simulink model "MDCC_DeadComp"  (R2023a)
settings: Solver=FixedStepDiscrete  StartTime=0.0  StopTime=10.0  FixedStep=0.0001  RelTol=1e-3
model workspace (MATLAB code in the model file):
  | cmdLim = Simulink.Parameter;
  | cmdLim.Value = 15;
  | cmdLim.Description = 'Limit for controlling the maximum surface command angle.';
  | cmdLim.Min = 0;
  | cmdLim.Max = 90;
  | cmdLim.DocUnits = 'deg';
  | 
  | dispGain = Simulink.Parameter;
  | dispGain.Value = 0.75;
  | dispGain.Description = 'Gain applied to the displacement error.';
  | dispGain.Min = 0;
  | dispGain.Max = [];
  | dispGain.DocUnits = 'deg/sec/deg';
  | 
  | dispLim = Simulink.Parameter;
  | dispLim.Value = 30;
  | dispLim.Description = 'Limit for controlling the maximum commanded angle.';
  | dispLim.Min = 0;
  | dispLim.Max = 180;
  | dispLim.DocUnits = 'deg';
  | 
  | intGain = Simulink.Parameter;
  | intGain.Value = 0.5;
  | intGain.Description = 'Gain applied to the integral error.';
  | intGain.Min = 0;
  | intGain.Max = [];
  | intGain.DocUnits = 'deg/sec/deg/sec';
  | 
  | intLim = Simulink.Parameter;
  | intLim.Value = 5;
  | intLim.Description = 'Limit for controlling the maximum commanded angle.';
  | intLim.Min = 0;
  | intLim.Max = 90;
  | intLim.DocUnits = 'deg';
  | 
  | rateGain = Simulink.Parameter;
  | rateGain.Value = 2;
  | rateGain.Description = 'Gain applied to the rate error.';
  | rateGain.Min = 0;
  | rateGain.Max = [];
  | rateGain.DocUnits = 'deg/deg/sec';
  | 
  | rateLim = Simulink.Parameter;
  | rateLim.Value = 6;
  | rateLim.Description = 'Limit for controlling the maximum commanded angle.';
  | rateLim.Min = 0;
  | rateLim.Max = 180;
  | rateLim.DocUnits = 'deg/sec';
  | 
  | hdgGain = Simulink.Parameter;
  | hdgGain.Value = 0.015;
values from neighbouring files (symbols this model uses):
  Ts = 5E-6    (= 5e-06)    [iPMSM_data.m]
undefined symbols (not defined in the file or in its folder): CosTable12bit_Y, GLBCal_GLBCal_Kf_DCLinkOverVolErrThd_V, GLBCal_GLBCal_Kf_DCLinkUnderVolErrThd_V, GLBCal_GLBCal_Kf_EquiLd_NULL, GLBCal_GLBCal_Kf_EquiLq_NULL, GLBCal_GLBCal_Kf_MotorRatedSpeed_rpm, GLBCal_GLBCal_Kf_MotorSpeedHysteresis_Coef, GLBCal_Ke_MotorPolePairsNum_NULL, IoHwAbOpArg_PwmDutyCyclePhU_NULL, IoHwAbOpArg_PwmDutyCyclePhV_NULL, IoHwAbOpArg_PwmDutyCyclePhW_NULL, IoHwAbOpArg_PwmOutputEn, KbMDCC_DeadTimeCompEn_flg, KbMDCC_MCF_flgHarmInject_flg, KbMDCC_SetEAngleEn_flg, KbMDCC_UdUqFwOmit_flg, KfMDCC_AbsIs_A, KfMDCC_ActiveDischargeIdCurVal_A, KfMDCC_ActiveDischargeIqCurVal_A, KfMDCC_DCLinkVolRate_coef, KfMDCC_DeadRate_NULL, KfMDCC_DebugEAngleInit_rad, KfMDCC_DebugUalphaVolCmd_V, KfMDCC_DebugUbetaVolCmd_V, KfMDCC_DebugUdCmd_V, KfMDCC_DebugUqCmd_V, KfMDCC_DebugUsCmd_V, KfMDCC_DebugUsRate_V, KfMDCC_Duty_Coef, KfMDCC_IMCResp_NULL, KfMDCC_IMCStab_NULL, KfMDCC_InvParkCpPeriodTimesT_NULL, KfMDCC_MCF_Harm1113FLParamSpeedThrd_rads, KfMDCC_MCF_Harm57FLParamSpeedThrd_rads, KfMDCC_MCF_HarmCpnAg_NULL, KfMDCC_MCF_HarmfLParaHigh_coef, KfMDCC_MCF_HarmfLParaLow_coef, KfMDCC_MCF_HarmInSpdLimt_rpm, KfMDCC_MCF_HarmInUAlphaMax_V, KfMDCC_MCF_HarmInUbetaMax_V, KfMDCC_MotorSpeedRadsDAQFactor_NULL, KfMDCC_ResScal_Coef, KfMDCC_SelfHeatingUdVal_V, KfMDCC_SelfHeatingUdValRate_V, KfMDCC_SpdIMCResp_rpm, KfMDCC_SpdIMCStab_rpm, KfMDCC_VfMDCC_DCLinkCurValFactor_NULL, KfMDCM_DCLinkCoef, KfMDCM_DCLinkRatedVoltage_V, KfMDCM_FluxWeakningVolFWOffset_V, KuMDCC_PositionResolution_NULL, KuMDCC_SetEAngle_Null, MDSM_MCUStatus, PiIoHwSetInvState_C_Sws_UVW_PwmEnOutput, PiIoHwSetInvState_C_SwsSet_DPO_UVW_Asc, PiIoHwSetInvState_C_SwsSet_DPO_UVW_FW, PiIoHwSetPwmDuty_C_SwsSet_DPO_UVW_Duty, SinTable12bit_Y, SVPWM, VfMDCC_DeadComSpeedHigh_Rpm ... (+5)
libraries: simulink x14, PMSM_Library x4
(part 4 of 6)

== system MDCC_DeadComp/DoCurCtr_sys/MDCC/SVM_Calc/MDSA/SVPWM1/vIntp_PWMFOC_CalSec/CalVaVbVc ==
  Bus_UalphaUbeta : Inport
  Bus Creator : BusCreator  Inputs=3
  CalVa : Subsystem
  CalVb : Subsystem
  CalVc : Subsystem
  Bus_Vabc : Outport
  wires:
  Bus_UalphaUbeta/1 -> CalVc/1(In1), CalVb/1(In1), CalVa/1(In1)
  CalVb/1(Vb) -> Bus Creator/2  "Vb"
  CalVc/1(Vc) -> Bus Creator/3  "Vc"
  CalVa/1(Va) -> Bus Creator/1  "Va"
  Bus Creator/1 -> Bus_Vabc/1

== system MDCC_DeadComp/DoCurCtr_sys/MDCC/SVM_Calc/MDSA/SVPWM1/vIntp_PWMFOC_CalTriCompValue/CalCMPValue ==
  Bus_Tabc_IN : Inport
  N_VALUE_IN : Inport  Port=2
  Merge : Merge  Inputs=6
  Sec1 : Subsystem
  Sec2 : Subsystem
  Sec3 : Subsystem
  Sec4 : Subsystem
  Sec5 : Subsystem
  Sec6 : Subsystem
  Switch Case : SwitchCase  CaseConditions={1,2,3,4,5,6}  ShowDefaultCase=off
  Bus_CMP : Outport
  wires:
  N_VALUE_IN/1 -> Switch Case/1
  Bus_Tabc_IN/1 -> Sec2/1(Bus_Tabc_IN), Sec4/1(Bus_Tabc_IN), Sec6/1(Bus_Tabc_IN), Sec5/1(Bus_Tabc_IN), Sec3/1(Bus_Tabc_IN), Sec1/1(Bus_Tabc_IN)
  Merge/1 -> Bus_CMP/1
  Switch Case/1 -> [sec1]
  Switch Case/2 -> [sec2]
  Switch Case/3 -> [sec3]
  Switch Case/4 -> [sec4]
  Switch Case/5 -> [sec5]
  Switch Case/6 -> [sec6]
  [sec1] -> Sec1/Action
  [sec2] -> Sec2/Action
  [sec3] -> Sec3/Action
  [sec4] -> Sec4/Action
  [sec5] -> Sec5/Action
  [sec6] -> Sec6/Action
  Sec4/1(Bus_CMP) -> Merge/4
  Sec3/1(Bus_CMP) -> Merge/3
  Sec5/1(Bus_CMP) -> Merge/5
  Sec2/1(Bus_CMP) -> Merge/2
  Sec6/1(Bus_CMP) -> Merge/6
  Sec1/1(Bus_CMP) -> Merge/1

== system MDCC_DeadComp/DoCurCtr_sys/MDCC/SVM_Calc/MDSA/SVPWM1/vIntp_PWMFOC_CalTriCompValue/CalTabc ==
  Bus_XYZ_IN : Inport
  Bus_Ts_Vdc : Inport  Port=2
  N_VALUE_IN : Inport  Port=3
  Cal_T1T2 : Subsystem
  Cal_TabcValue : Subsystem
  Bus_Tabc : Outport
  wires:
  Bus_Ts_Vdc/1 -> Cal_TabcValue/2(Bus_Ts_Vdc)
  Bus_XYZ_IN/1 -> Cal_T1T2/1(Bus_XYZ_IN)
  N_VALUE_IN/1 -> Cal_T1T2/2(N_VALUE_IN)
  Cal_T1T2/1(Bus_T1T2_OUT) -> Cal_TabcValue/1(Bus_T1T2_IN)
  Cal_TabcValue/1(Bus_Tabc) -> Bus_Tabc/1

== system MDCC_DeadComp/DoCurCtr_sys/MDCC/SVM_Calc/MDSA/SVPWM1/vIntp_PWMFOC_CalTriCompValue/CalXYZ ==
  Bus_UalphaUbeta : Inport
  Bus_Ts_Vdc : Inport  Port=2
  Bus Creator : BusCreator  Inputs=3
  Cal_X : Subsystem
  Cal_Y : Subsystem
  Cal_Z : Subsystem
  BUS_XYZ : Outport
  wires:
  Bus_UalphaUbeta/1 -> Cal_Z/1(Bus_UalphaUbeta), Cal_Y/1(Bus_UalphaUbeta), Cal_X/1(Bus_UalphaUbeta)
  Cal_Y/1(Y_Value) -> Bus Creator/2  "Y"
  Cal_X/1(X_Value) -> Bus Creator/1  "X"
  Cal_Z/1(Z_Value) -> Bus Creator/3  "Z"
  Bus Creator/1 -> BUS_XYZ/1
  Bus_Ts_Vdc/1 -> Cal_Z/2(Bus_Ts_Vdc), Cal_X/2(Bus_Ts_Vdc), Cal_Y/2(Bus_Ts_Vdc)

== system MDCC_DeadComp/DoCurCtr_sys/MDCC/UdUqCalc_Sys/MDCC_MCF_Sys1/Enabled Subsystem/Harmonic_Injection_11/Subsystem ==
  MCF_Harm_isdDes11 : Inport
  MCF_Harm_isqDes11 : Inport  Port=2
  MCF_Harm_isdAct11 : Inport  Port=3
  MCF_Harm_isqAct11 : Inport  Port=4
  MCF_Sin11Ag : Inport  Port=5
  MCF_Cos11Ag : Inport  Port=6
  MCF_flgHarm11PIRest : Inport  Port=7
  MCF_Harm11_Kp : Inport  Port=8
  MCF_Harm11_Ki : Inport  Port=9
  ZeroEnable : EnablePort  StatesWhenEnabling=reset
  Harm_11Step_KpKi : Subsystem
  RevPark : Subsystem
  MCF_uAlpha_Harm11 : Outport  VectorParamsAs1DForOutWhenUnconnected=off
  MCF_uBeta_Harm11 : Outport  Port=2  VectorParamsAs1DForOutWhenUnconnected=off
  wires:
  MCF_Harm_isqDes11/1 -> Harm_11Step_KpKi/2(MCF_Harm_isqDes11)  "MCF_Harm_isqDes11"
  MCF_Harm_isqAct11/1 -> Harm_11Step_KpKi/4(MCF_Harm_isqAct11)
  RevPark/2(MCF_uBeta_Harm11) -> MCF_uBeta_Harm11/1
  MCF_Harm_isdAct11/1 -> Harm_11Step_KpKi/3(MCF_Harm_isdAct11)
  RevPark/1(MCF_uAlpha_Harm11) -> MCF_uAlpha_Harm11/1
  MCF_Harm_isdDes11/1 -> Harm_11Step_KpKi/1(MCF_Harm_isdDes11)  "MCF_Harm_isdDes11"
  MCF_flgHarm11PIRest/1 -> Harm_11Step_KpKi/5(MCF_flgHarm11PIRest)
  Harm_11Step_KpKi/1(MCF_Harm_ud11PI) -> RevPark/1(MCF_Harm_ud11PI)
  Harm_11Step_KpKi/2(MCF_Harm_uq11PI) -> RevPark/2(MCF_Harm_uq11PI)
  MCF_Sin11Ag/1 -> RevPark/3(MCF_Sin11Ag)
  MCF_Cos11Ag/1 -> RevPark/4(MCF_Cos11Ag)
  MCF_Harm11_Kp/1 -> Harm_11Step_KpKi/6(MCF_Harm11_Kp)
  MCF_Harm11_Ki/1 -> Harm_11Step_KpKi/7(MCF_Harm11_Ki)

== system MDCC_DeadComp/DoCurCtr_sys/MDCC/UdUqCalc_Sys/MDCC_MCF_Sys1/Enabled Subsystem/Harmonic_Injection_13/Subsystem ==
  MCF_Harm_isdDes13 : Inport
  MCF_Harm_isqDes13 : Inport  Port=2
  MCF_Harm_isdAct13 : Inport  Port=3
  MCF_Harm_isqAct13 : Inport  Port=4
  MCF_Sin13Ag : Inport  Port=5
  MCF_Cos13Ag : Inport  Port=6
  MCF_flgHarm13PIRest : Inport  Port=7
  MCF_Harm13_Kp : Inport  Port=8
  MCF_Harm13_Ki : Inport  Port=9
  ZeroEnable : EnablePort  StatesWhenEnabling=reset
  Harm_13Step_KpKi : Subsystem
  RevPark : Subsystem
  MCF_uAlpha_Harm13 : Outport  VectorParamsAs1DForOutWhenUnconnected=off
  MCF_uBeta_Harm13 : Outport  Port=2  VectorParamsAs1DForOutWhenUnconnected=off
  wires:
  MCF_Harm_isqDes13/1 -> Harm_13Step_KpKi/2(MCF_Harm_isqDes13)  "MCF_Harm_isqDes13"
  MCF_Harm_isqAct13/1 -> Harm_13Step_KpKi/4(MCF_Harm_isqAct13)
  RevPark/2(MCF_uBeta_Harm13) -> MCF_uBeta_Harm13/1
  MCF_Harm_isdAct13/1 -> Harm_13Step_KpKi/3(MCF_Harm_isdAct13)
  RevPark/1(MCF_uAlpha_Harm13) -> MCF_uAlpha_Harm13/1
  MCF_Harm_isdDes13/1 -> Harm_13Step_KpKi/1(MCF_Harm_isdDes13)  "MCF_Harm_isdDes13"
  MCF_flgHarm13PIRest/1 -> Harm_13Step_KpKi/5(MCF_flgHarm13PIRest)
  Harm_13Step_KpKi/1(MCF_Harm_ud13PI) -> RevPark/1(MCF_Harm_ud13PI)
  Harm_13Step_KpKi/2(MCF_Harm_uq13PI) -> RevPark/2(MCF_Harm_uq13PI)
  MCF_Sin13Ag/1 -> RevPark/3(MCF_Sin13Ag)
  MCF_Cos13Ag/1 -> RevPark/4(MCF_Cos13Ag)
  MCF_Harm13_Kp/1 -> Harm_13Step_KpKi/6(MCF_Harm13_Kp)
  MCF_Harm13_Ki/1 -> Harm_13Step_KpKi/7(MCF_Harm13_Ki)

== system MDCC_DeadComp/DoCurCtr_sys/MDCC/UdUqCalc_Sys/MDCC_MCF_Sys1/Enabled Subsystem/Harmonic_Injection_5/Subsystem ==
  MCF_Harm_isdDes5 : Inport
  MCF_Harm_isqDes5 : Inport  Port=2
  MCF_Harm_isdAct5 : Inport  Port=3
  MCF_Harm_isqAct5 : Inport  Port=4
  MCF_Sin5Ag : Inport  Port=5
  MCF_Cos5Ag : Inport  Port=6
  MCF_flgHarm5PIRest : Inport  Port=7
  MCF_Harm5_Kp : Inport  Port=8
  MCF_Harm5_Ki : Inport  Port=9
  ZeroEnable : EnablePort  StatesWhenEnabling=reset
  Harm_5Step_KpKi : Subsystem
  RevPark : Subsystem
  MCF_uAlpha_Harm5 : Outport  VectorParamsAs1DForOutWhenUnconnected=off
  MCF_uBeta_Harm5 : Outport  Port=2  VectorParamsAs1DForOutWhenUnconnected=off
  wires:
  MCF_Harm_isqDes5/1 -> Harm_5Step_KpKi/2(MCF_Harm_isqDes5)  "MCF_Harm_isqDes5"
  MCF_Harm_isqAct5/1 -> Harm_5Step_KpKi/4(MCF_Harm_isqAct5)
  RevPark/2(MCF_uBeta_Harm5) -> MCF_uBeta_Harm5/1
  MCF_Harm_isdAct5/1 -> Harm_5Step_KpKi/3(MCF_Harm_isdAct5)
  RevPark/1(MCF_uAlpha_Harm5) -> MCF_uAlpha_Harm5/1
  MCF_Harm_isdDes5/1 -> Harm_5Step_KpKi/1(MCF_Harm_isdDes5)  "MCF_Harm_isdDes5"
  MCF_flgHarm5PIRest/1 -> Harm_5Step_KpKi/5(MCF_flgHarm5PIRest)
  Harm_5Step_KpKi/1(MCF_Harm_ud5PI) -> RevPark/1(MCF_Harm_ud5PI)
  Harm_5Step_KpKi/2(MCF_Harm_uq5PI) -> RevPark/2(MCF_Harm_uq5PI)
  MCF_Sin5Ag/1 -> RevPark/3(MCF_Sin5Ag)
  MCF_Cos5Ag/1 -> RevPark/4(MCF_Cos5Ag)
  MCF_Harm5_Kp/1 -> Harm_5Step_KpKi/6(MCF_Harm5_Kp)
  MCF_Harm5_Ki/1 -> Harm_5Step_KpKi/7(MCF_Harm5_Ki)

== system MDCC_DeadComp/DoCurCtr_sys/MDCC/UdUqCalc_Sys/MDCC_MCF_Sys1/Enabled Subsystem/Harmonic_Injection_7/Subsystem ==
  MCF_Harm_isdDes7 : Inport
  MCF_Harm_isqDes7 : Inport  Port=2
  MCF_Harm_isdAct7 : Inport  Port=3
  MCF_Harm_isqAct7 : Inport  Port=4
  MCF_Sin7Ag : Inport  Port=5
  MCF_Cos7Ag : Inport  Port=6
  MCF_flgHarm7PIRest : Inport  Port=7
  MCF_Harm7_Kp : Inport  Port=8
  MCF_Harm7_Ki : Inport  Port=9
  ZeroEnable : EnablePort  StatesWhenEnabling=reset
  Harm_7Step_KpKi : Subsystem
  RevPark : Subsystem
  MCF_uAlpha_Harm7 : Outport  VectorParamsAs1DForOutWhenUnconnected=off
  MCF_uBeta_Harm7 : Outport  Port=2  VectorParamsAs1DForOutWhenUnconnected=off
  wires:
  MCF_Harm_isqDes7/1 -> Harm_7Step_KpKi/2(MCF_Harm_isqDes7)  "MCF_Harm_isqDes7"
  MCF_Harm_isqAct7/1 -> Harm_7Step_KpKi/4(MCF_Harm_isqAct7)
  RevPark/2(MCF_uBeta_Harm7) -> MCF_uBeta_Harm7/1
  MCF_Harm_isdAct7/1 -> Harm_7Step_KpKi/3(MCF_Harm_isdAct7)
  RevPark/1(MCF_uAlpha_Harm7) -> MCF_uAlpha_Harm7/1
  MCF_Harm_isdDes7/1 -> Harm_7Step_KpKi/1(MCF_Harm_isdDes7)  "MCF_Harm_isdDes7"
  MCF_flgHarm7PIRest/1 -> Harm_7Step_KpKi/5(MCF_flgHarm7PIRest)
  Harm_7Step_KpKi/1(MCF_Harm_ud7PI) -> RevPark/1(MCF_Harm_ud7PI)
  Harm_7Step_KpKi/2(MCF_Harm_uq7PI) -> RevPark/2(MCF_Harm_uq7PI)
  MCF_Sin7Ag/1 -> RevPark/3(MCF_Sin7Ag)
  MCF_Cos7Ag/1 -> RevPark/4(MCF_Cos7Ag)
  MCF_Harm7_Kp/1 -> Harm_7Step_KpKi/6(MCF_Harm7_Kp)
  MCF_Harm7_Ki/1 -> Harm_7Step_KpKi/7(MCF_Harm7_Ki)

== system MDCC_DeadComp/DoCurCtr_sys/MDCC/UdUqCalc_Sys/MDCC_MCF_Sys1/Enabled Subsystem/Subsystem1/Park11 ==
  note: 低通滤波器
  MCF_AgSin : Inport
  MCF_ialpha_Harm : Inport  Port=2
  MCF_ibeta_Harm : Inport  Port=3
  MCF_AgCos : Inport  Port=4
  MCF_dtPWM : Inport  Port=5
  dB_Harm : Inport  Port=6
  Add : Sum
  Add1 : Sum  Inputs=-+
  Product{,1..3} (4 alike) : Product
  Subsystem : Subsystem
  Subsystem1 : Subsystem
  MCF_Id_Harm : Outport
  MCF_Iq_Harm : Outport  Port=2
  wires:
  Add/1 -> Subsystem/1(In1)
  Add1/1 -> Subsystem1/3(In1)
  Product2/1 -> Add1/1
  Product/1 -> Add/1
  Product1/1 -> Add/2
  Product3/1 -> Add1/2
  Subsystem/1(Out1) -> MCF_Id_Harm/1  "MCF_Id11_Harm"
  Subsystem1/1(Out1) -> MCF_Iq_Harm/1  "MCF_Iq11_Harm"
  MCF_ialpha_Harm/1 -> Product2/1, Product/1
  MCF_AgCos/1 -> Product/2, Product3/2
  MCF_ibeta_Harm/1 -> Product1/1, Product3/1
  MCF_AgSin/1 -> Product1/2, Product2/2
  MCF_dtPWM/1 -> Subsystem1/2(MCF_dtPWM), Subsystem/2(MCF_dtPWM)
  dB_Harm/1 -> Subsystem/3(dB_Harm), Subsystem1/1(dB_Harm)

== system MDCC_DeadComp/DoCurCtr_sys/MDCC/UdUqCalc_Sys/MDCC_MCF_Sys1/Enabled Subsystem/Subsystem1/Park13 ==
  note: 低通滤波器
  MCF_AgSin : Inport
  MCF_ialpha_Harm : Inport  Port=2
  MCF_ibeta_Harm : Inport  Port=3
  MCF_AgCos : Inport  Port=4
  MCF_dtPWM : Inport  Port=5
  dB_Harm : Inport  Port=6
  Add : Sum
  Add1 : Sum  Inputs=-+
  Product{,1..3} (4 alike) : Product
  Subsystem : Subsystem
  Subsystem1 : Subsystem
  MCF_Id_Harm : Outport
  MCF_Iq_Harm : Outport  Port=2
  wires:
  Add/1 -> Subsystem/1(In1)
  Add1/1 -> Subsystem1/3(In1)
  Product2/1 -> Add1/1
  Product/1 -> Add/1
  Product1/1 -> Add/2
  Product3/1 -> Add1/2
  Subsystem/1(Out1) -> MCF_Id_Harm/1  "MCF_Id13_Harm"
  Subsystem1/1(Out1) -> MCF_Iq_Harm/1  "MCF_Iq13_Harm"
  MCF_ialpha_Harm/1 -> Product2/1, Product/1
  MCF_AgCos/1 -> Product/2, Product3/2
  MCF_ibeta_Harm/1 -> Product1/1, Product3/1
  MCF_AgSin/1 -> Product1/2, Product2/2
  MCF_dtPWM/1 -> Subsystem1/2(MCF_dtPWM), Subsystem/2(MCF_dtPWM)
  dB_Harm/1 -> Subsystem/3(dB_Harm), Subsystem1/1(dB_Harm)

== system MDCC_DeadComp/DoCurCtr_sys/MDCC/UdUqCalc_Sys/MDCC_MCF_Sys1/Enabled Subsystem/Subsystem1/Park5 ==
  note: 低通滤波器
  MCF_AgSin : Inport
  MCF_ialpha_Harm : Inport  Port=2
  MCF_ibeta_Harm : Inport  Port=3
  MCF_AgCos : Inport  Port=4
  MCF_dtPWM : Inport  Port=5
  dB_Harm : Inport  Port=6
  Add : Sum
  Add1 : Sum  Inputs=-+
  Product{,1..3} (4 alike) : Product
  Subsystem : Subsystem
  Subsystem1 : Subsystem
  MCF_Id_Harm : Outport
  MCF_Iq_Harm : Outport  Port=2
  wires:
  Add/1 -> Subsystem/1(In1)
  Add1/1 -> Subsystem1/3(In1)
  Product2/1 -> Add1/1
  Product/1 -> Add/1
  Product1/1 -> Add/2
  Product3/1 -> Add1/2
  Subsystem/1(Out1) -> MCF_Id_Harm/1  "MCF_Id5_Harm"
  Subsystem1/1(Out1) -> MCF_Iq_Harm/1  "MCF_Iq5_Harm"
  MCF_ialpha_Harm/1 -> Product2/1, Product/1
  MCF_AgCos/1 -> Product/2, Product3/2
  MCF_ibeta_Harm/1 -> Product1/1, Product3/1
  MCF_AgSin/1 -> Product1/2, Product2/2
  MCF_dtPWM/1 -> Subsystem1/2(MCF_dtPWM), Subsystem/2(MCF_dtPWM)
  dB_Harm/1 -> Subsystem/3(dB_Harm), Subsystem1/1(dB_Harm)

== system MDCC_DeadComp/DoCurCtr_sys/MDCC/UdUqCalc_Sys/MDCC_MCF_Sys1/Enabled Subsystem/Subsystem1/Park7 ==
  note: 低通滤波器
  MCF_AgSin : Inport
  MCF_ialpha_Harm : Inport  Port=2
  MCF_ibeta_Harm : Inport  Port=3
  MCF_AgCos : Inport  Port=4
  MCF_dtPWM : Inport  Port=5
  dB_Harm : Inport  Port=6
  Add : Sum
  Add1 : Sum  Inputs=-+
  Product{,1..3} (4 alike) : Product
  Subsystem : Subsystem
  Subsystem1 : Subsystem
  MCF_Id_Harm : Outport
  MCF_Iq_Harm : Outport  Port=2
  wires:
  Add/1 -> Subsystem/1(In1)
  Add1/1 -> Subsystem1/3(In1)
  Product2/1 -> Add1/1
  Product/1 -> Add/1
  Product1/1 -> Add/2
  Product3/1 -> Add1/2
  Subsystem/1(Out1) -> MCF_Id_Harm/1  "MCF_Id7_Harm"
  Subsystem1/1(Out1) -> MCF_Iq_Harm/1  "MCF_Iq7_Harm"
  MCF_ialpha_Harm/1 -> Product2/1, Product/1
  MCF_AgCos/1 -> Product/2, Product3/2
  MCF_ibeta_Harm/1 -> Product1/1, Product3/1
  MCF_AgSin/1 -> Product1/2, Product2/2
  MCF_dtPWM/1 -> Subsystem1/2(MCF_dtPWM), Subsystem/2(MCF_dtPWM)
  dB_Harm/1 -> Subsystem/3(dB_Harm), Subsystem1/1(dB_Harm)

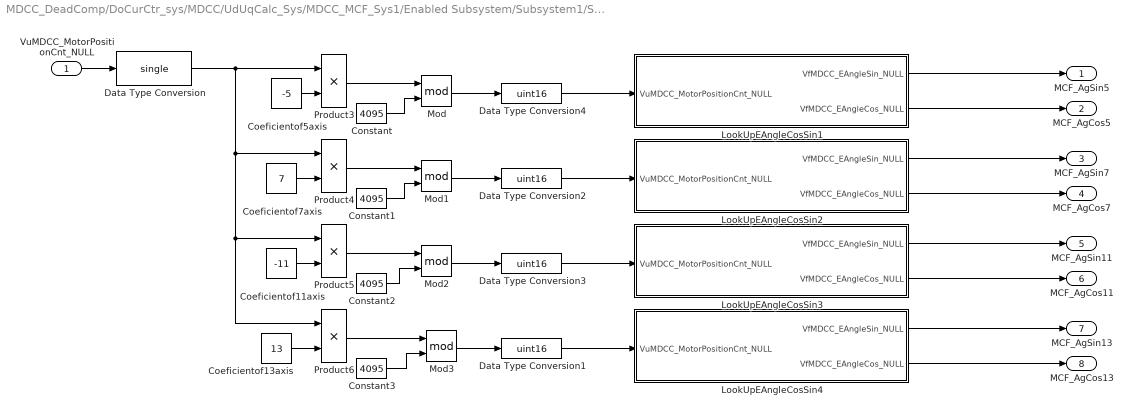
== system MDCC_DeadComp/DoCurCtr_sys/MDCC/UdUqCalc_Sys/MDCC_MCF_Sys1/Enabled Subsystem/Subsystem1/Subsystem ==
  VuMDCC_MotorPositionCnt_NULL : Inport
  Coeficientof11axis : Constant  Value=-11  OutDataTypeStr=single
  Coeficientof13axis : Constant  Value=13  OutDataTypeStr=single
  Coeficientof5axis : Constant  Value=-5  OutDataTypeStr=single
  Coeficientof7axis : Constant  Value=7  OutDataTypeStr=single
  Constant{,1..3} (4 alike) : Constant  Value=4095  OutDataTypeStr=single
  Data Type Conversion : DataTypeConversion  OutDataTypeStr=single  SaturateOnIntegerOverflow=off  RndMeth=Floor
  Data Type Conversion{1..4} (4 alike) : DataTypeConversion  OutDataTypeStr=uint16  SaturateOnIntegerOverflow=off  RndMeth=Floor
  LookUpEAngleCosSin1 : Subsystem  TreatAsAtomicUnit=on  RTWFcnName=MCF_MDCC_LookUpEAngleCosSin  RTWFileName=MDCC
      settings: RTWFcnNameOpts=User specified
  LookUpEAngleCosSin2 : Subsystem  TreatAsAtomicUnit=on  RTWFcnName=MCF_MDCC_LookUpEAngleCosSin  RTWFileName=MDCC
      settings: RTWFcnNameOpts=User specified
  LookUpEAngleCosSin3 : Subsystem  TreatAsAtomicUnit=on  RTWFcnName=MCF_MDCC_LookUpEAngleCosSin  RTWFileName=MDCC
      settings: RTWFcnNameOpts=User specified
  LookUpEAngleCosSin4 : Subsystem  TreatAsAtomicUnit=on  RTWFcnName=MCF_MDCC_LookUpEAngleCosSin  RTWFileName=MDCC
      settings: RTWFcnNameOpts=User specified
  Mod{,1..3} (4 alike) : Math  Operator=mod
  Product{3..6} (4 alike) : Product
  MCF_AgSin5 : Outport
  MCF_AgCos5 : Outport  Port=2
  MCF_AgSin7 : Outport  Port=3
  MCF_AgCos7 : Outport  Port=4
  MCF_AgSin11 : Outport  Port=5
  MCF_AgCos11 : Outport  Port=6
  MCF_AgSin13 : Outport  Port=7
  MCF_AgCos13 : Outport  Port=8
  wires:
  Coeficientof5axis/1 -> Product3/2
  LookUpEAngleCosSin1/1(VfMDCC_EAngleSin_NULL) -> MCF_AgSin5/1
  LookUpEAngleCosSin1/2(VfMDCC_EAngleCos_NULL) -> MCF_AgCos5/1
  Coeficientof7axis/1 -> Product4/2
  LookUpEAngleCosSin2/2(VfMDCC_EAngleCos_NULL) -> MCF_AgCos7/1
  LookUpEAngleCosSin2/1(VfMDCC_EAngleSin_NULL) -> MCF_AgSin7/1
  Coeficientof11axis/1 -> Product5/2
  LookUpEAngleCosSin3/2(VfMDCC_EAngleCos_NULL) -> MCF_AgCos11/1
  LookUpEAngleCosSin3/1(VfMDCC_EAngleSin_NULL) -> MCF_AgSin11/1
  Coeficientof13axis/1 -> Product6/2
  VuMDCC_MotorPositionCnt_NULL/1 -> Data Type Conversion/1
  LookUpEAngleCosSin4/1(VfMDCC_EAngleSin_NULL) -> MCF_AgSin13/1
  LookUpEAngleCosSin4/2(VfMDCC_EAngleCos_NULL) -> MCF_AgCos13/1
  Data Type Conversion/1 -> Product6/1, Product5/1, Product4/1, Product3/1
  Constant/1 -> Mod/2
  Constant1/1 -> Mod1/2
  Constant2/1 -> Mod2/2
  Constant3/1 -> Mod3/2
  Product4/1 -> Mod1/1
  Product6/1 -> Mod3/1
  Product5/1 -> Mod2/1
  Product3/1 -> Mod/1
  Mod1/1 -> Data Type Conversion2/1
  Mod/1 -> Data Type Conversion4/1
  Mod2/1 -> Data Type Conversion3/1
  Mod3/1 -> Data Type Conversion1/1
  Data Type Conversion1/1 -> LookUpEAngleCosSin4/1(VuMDCC_MotorPositionCnt_NULL)
  Data Type Conversion3/1 -> LookUpEAngleCosSin3/1(VuMDCC_MotorPositionCnt_NULL)
  Data Type Conversion2/1 -> LookUpEAngleCosSin2/1(VuMDCC_MotorPositionCnt_NULL)
  Data Type Conversion4/1 -> LookUpEAngleCosSin1/1(VuMDCC_MotorPositionCnt_NULL)

== system MDCC_DeadComp/DoCurCtr_sys/MDCC/UdUqCalc_Sys/MDCC_MCF_Sys1/Enabled Subsystem/Subsystem2/Mcf_AgTranCalc1 ==
  Harm_AgCpn : Inport
  Harm_coef : Inport  Port=2
  Constant : Constant  Value=4095  OutDataTypeStr=single
  Data Type Conversion : DataTypeConversion  OutDataTypeStr=uint16  SaturateOnIntegerOverflow=off  RndMeth=Floor
  Divide2 : Product  Inputs=**  OutDataTypeStr=single
  LookUpEAngleCosSin2 : Subsystem  TreatAsAtomicUnit=on  RTWFcnName=MCF_MDCC_LookUpEAngleCosSin  RTWFileName=MDCC
      settings: RTWFcnNameOpts=User specified
  Mod : Math  Operator=mod
  MCF_SinAg : Outport  VectorParamsAs1DForOutWhenUnconnected=off
  MCF_CosAg : Outport  Port=2  VectorParamsAs1DForOutWhenUnconnected=off
  wires:
  Data Type Conversion/1 -> LookUpEAngleCosSin2/1(VuMDCC_MotorPositionCnt_NULL)
  Mod/1 -> Data Type Conversion/1
  Harm_coef/1 -> Divide2/2
  Constant/1 -> Mod/2
  Divide2/1 -> Mod/1
  Harm_AgCpn/1 -> Divide2/1
  LookUpEAngleCosSin2/1(VfMDCC_EAngleSin_NULL) -> MCF_SinAg/1  "MCF_SinAg"
  LookUpEAngleCosSin2/2(VfMDCC_EAngleCos_NULL) -> MCF_CosAg/1  "MCF_CosAg"

== system MDCC_DeadComp/DoCurCtr_sys/MDCC/UdUqCalc_Sys/MDCC_MCF_Sys1/Enabled Subsystem/Subsystem2/Mcf_AgTranCalc2 ==
  Harm_AgCpn : Inport
  Harm_coef : Inport  Port=2
  Constant : Constant  Value=4095  OutDataTypeStr=single
  Data Type Conversion : DataTypeConversion  OutDataTypeStr=uint16  SaturateOnIntegerOverflow=off  RndMeth=Floor
  Divide2 : Product  Inputs=**  OutDataTypeStr=single
  LookUpEAngleCosSin2 : Subsystem  TreatAsAtomicUnit=on  RTWFcnName=MCF_MDCC_LookUpEAngleCosSin  RTWFileName=MDCC
      settings: RTWFcnNameOpts=User specified
  Mod : Math  Operator=mod
  MCF_SinAg : Outport  VectorParamsAs1DForOutWhenUnconnected=off
  MCF_CosAg : Outport  Port=2  VectorParamsAs1DForOutWhenUnconnected=off
  wires:
  LookUpEAngleCosSin2/2(VfMDCC_EAngleCos_NULL) -> MCF_CosAg/1  "MCF_CosAg"
  LookUpEAngleCosSin2/1(VfMDCC_EAngleSin_NULL) -> MCF_SinAg/1  "MCF_SinAg"
  Harm_AgCpn/1 -> Divide2/1
  Divide2/1 -> Mod/1
  Constant/1 -> Mod/2
  Harm_coef/1 -> Divide2/2
  Mod/1 -> Data Type Conversion/1
  Data Type Conversion/1 -> LookUpEAngleCosSin2/1(VuMDCC_MotorPositionCnt_NULL)

== system MDCC_DeadComp/DoCurCtr_sys/MDCC/UdUqCalc_Sys/MDCC_MCF_Sys1/Enabled Subsystem/Subsystem2/Mcf_AgTranCalc3 ==
  Harm_AgCpn : Inport
  Harm_coef : Inport  Port=2
  Constant : Constant  Value=4095  OutDataTypeStr=single
  Data Type Conversion : DataTypeConversion  OutDataTypeStr=uint16  SaturateOnIntegerOverflow=off  RndMeth=Floor
  Divide2 : Product  Inputs=**  OutDataTypeStr=single
  LookUpEAngleCosSin2 : Subsystem  TreatAsAtomicUnit=on  RTWFcnName=MCF_MDCC_LookUpEAngleCosSin  RTWFileName=MDCC
      settings: RTWFcnNameOpts=User specified
  Mod : Math  Operator=mod
  MCF_SinAg : Outport  VectorParamsAs1DForOutWhenUnconnected=off
  MCF_CosAg : Outport  Port=2  VectorParamsAs1DForOutWhenUnconnected=off
  wires:
  Data Type Conversion/1 -> LookUpEAngleCosSin2/1(VuMDCC_MotorPositionCnt_NULL)
  Mod/1 -> Data Type Conversion/1
  Harm_coef/1 -> Divide2/2
  Constant/1 -> Mod/2
  Divide2/1 -> Mod/1
  Harm_AgCpn/1 -> Divide2/1
  LookUpEAngleCosSin2/1(VfMDCC_EAngleSin_NULL) -> MCF_SinAg/1  "MCF_SinAg"
  LookUpEAngleCosSin2/2(VfMDCC_EAngleCos_NULL) -> MCF_CosAg/1  "MCF_CosAg"

== system MDCC_DeadComp/DoCurCtr_sys/MDCC/UdUqCalc_Sys/MDCC_MCF_Sys1/Enabled Subsystem/Subsystem2/Mcf_AgTranCalc5 ==
  Harm_AgCpn : Inport
  Harm_coef : Inport  Port=2
  Constant : Constant  Value=4095  OutDataTypeStr=single
  Data Type Conversion : DataTypeConversion  OutDataTypeStr=uint16  SaturateOnIntegerOverflow=off  RndMeth=Floor
  Divide2 : Product  Inputs=**  OutDataTypeStr=single
  LookUpEAngleCosSin2 : Subsystem  TreatAsAtomicUnit=on  RTWFcnName=MCF_MDCC_LookUpEAngleCosSin  RTWFileName=MDCC
      settings: RTWFcnNameOpts=User specified
  Mod : Math  Operator=mod
  MCF_SinAg : Outport  VectorParamsAs1DForOutWhenUnconnected=off
  MCF_CosAg : Outport  Port=2  VectorParamsAs1DForOutWhenUnconnected=off
  wires:
  LookUpEAngleCosSin2/2(VfMDCC_EAngleCos_NULL) -> MCF_CosAg/1  "MCF_CosAg"
  LookUpEAngleCosSin2/1(VfMDCC_EAngleSin_NULL) -> MCF_SinAg/1  "MCF_SinAg"
  Harm_AgCpn/1 -> Divide2/1
  Divide2/1 -> Mod/1
  Constant/1 -> Mod/2
  Harm_coef/1 -> Divide2/2
  Mod/1 -> Data Type Conversion/1
  Data Type Conversion/1 -> LookUpEAngleCosSin2/1(VuMDCC_MotorPositionCnt_NULL)

== system MDCC_DeadComp/DoCurCtr_sys/MDCC/UdUqCalc_Sys/MDCC_MCF_Sys1/Enabled Subsystem/Subsystem2/Subsystem ==
  HSPF_nSlowFlt : Inport
  dtPwmWoRpwm : Inport  Port=2
  MCF_agRtrEe : Inport  Port=3
  Add : Sum
  CAL_MCF_Harm_CpnAg_f32 : Constant  Value=KfMDCC_MCF_HarmCpnAg_NULL
  Constant : Constant  Value=4095  OutDataTypeStr=single
  Data Type Conversion : DataTypeConversion  OutDataTypeStr=single  SaturateOnIntegerOverflow=off  RndMeth=Floor
  Gain : Gain  Gain=4095/(2*pi)  OutDataTypeStr=single
  Mod : Math  Operator=mod
  Product1 : Product
  Product2 : Product
  Harm_AgCpn : Outport
  wires:
  CAL_MCF_Harm_CpnAg_f32/1 -> Product1/2
  HSPF_nSlowFlt/1 -> Product2/1
  dtPwmWoRpwm/1 -> Product2/2
  Product2/1 -> Product1/1
  Product1/1 -> Gain/1
  Add/1 -> Mod/1
  MCF_agRtrEe/1 -> Data Type Conversion/1
  Gain/1 -> Add/1
  Mod/1 -> Harm_AgCpn/1  "Harm_AgCpn"
  Constant/1 -> Mod/2
  Data Type Conversion/1 -> Add/2

== system MDCC_DeadComp/DoCurCtr_sys/MDCC/UdUqCalc_Sys/SelfHeating/Subsystem1/Subsystem1/Subsystem1 ==
  set : Inport
  rate : Inport  Port=2
  this_ref : Inport  Port=3
  Add : Sum  OutDataTypeStr=single
  Data Type Conversion : DataTypeConversion  OutDataTypeStr=single  SaturateOnIntegerOverflow=off  RndMeth=Floor
  MinMax : MinMax  Inputs=2  OutDataTypeStr=single
  MinMax1 : MinMax  Function=max  Inputs=2
  Subtract : Sum  Inputs=+-
  VfMDTM_SelfHeatingUdVal_V : Outport
  wires:
  rate/1 -> Subtract/2, Add/2
  MinMax1/1 -> VfMDTM_SelfHeatingUdVal_V/1
  this_ref/1 -> Subtract/1, Add/1
  set/1 -> Data Type Conversion/1
  Add/1 -> MinMax/2
  Subtract/1 -> MinMax1/2
  MinMax/1 -> MinMax1/1
  Data Type Conversion/1 -> MinMax/1

== system MDCC_DeadComp/DoCurCtr_sys/MDCC/SVM_Calc/MDSA/SVPWM1/vIntp_PWMFOC_CalSec/CalABC/CalA ==
  In1 : Inport
  Constant : Constant
  Constant1 : Constant  Value=0
  Data Type Conversion : DataTypeConversion  SaturateOnIntegerOverflow=off  RndMeth=Floor
  Data Type Conversion1 : DataTypeConversion  SaturateOnIntegerOverflow=off  RndMeth=Floor
  Switch : Switch  Criteria=u2 > Threshold  ZeroCross=off  SaturateOnIntegerOverflow=off  InputSameDT=off
  A : Outport
  wires:
  In1/1 -> Switch/2
  Constant/1 -> Data Type Conversion/1
  Constant1/1 -> Data Type Conversion1/1
  Data Type Conversion/1 -> Switch/1
  Data Type Conversion1/1 -> Switch/3
  Switch/1 -> A/1

== system MDCC_DeadComp/DoCurCtr_sys/MDCC/SVM_Calc/MDSA/SVPWM1/vIntp_PWMFOC_CalSec/CalABC/CalB ==
  In1 : Inport
  Constant : Constant
  Constant1 : Constant  Value=0
  Data Type Conversion : DataTypeConversion  SaturateOnIntegerOverflow=off  RndMeth=Floor
  Data Type Conversion1 : DataTypeConversion  SaturateOnIntegerOverflow=off  RndMeth=Floor
  Switch : Switch  Criteria=u2 > Threshold  ZeroCross=off  SaturateOnIntegerOverflow=off  InputSameDT=off
  B : Outport
  wires:
  Switch/1 -> B/1
  Data Type Conversion1/1 -> Switch/3
  Data Type Conversion/1 -> Switch/1
  Constant1/1 -> Data Type Conversion1/1
  Constant/1 -> Data Type Conversion/1
  In1/1 -> Switch/2

== system MDCC_DeadComp/DoCurCtr_sys/MDCC/SVM_Calc/MDSA/SVPWM1/vIntp_PWMFOC_CalSec/CalABC/CalC ==
  In1 : Inport
  Constant : Constant
  Constant1 : Constant  Value=0
  Data Type Conversion : DataTypeConversion  SaturateOnIntegerOverflow=off  RndMeth=Floor
  Data Type Conversion1 : DataTypeConversion  SaturateOnIntegerOverflow=off  RndMeth=Floor
  Switch : Switch  Criteria=u2 > Threshold  ZeroCross=off  SaturateOnIntegerOverflow=off  InputSameDT=off
  C : Outport
  wires:
  In1/1 -> Switch/2
  Constant/1 -> Data Type Conversion/1
  Constant1/1 -> Data Type Conversion1/1
  Data Type Conversion/1 -> Switch/1
  Data Type Conversion1/1 -> Switch/3
  Switch/1 -> C/1

== system MDCC_DeadComp/DoCurCtr_sys/MDCC/SVM_Calc/MDSA/SVPWM1/vIntp_PWMFOC_CalSec/CalVaVbVc/CalVa ==
  In1 : Inport
  Bus Selector : BusSelector  OutputSignals=Ubeta
  Va : Outport
  wires:
  In1/1 -> Bus Selector/1
  Bus Selector/1 -> Va/1  "<Ubeta>"

== system MDCC_DeadComp/DoCurCtr_sys/MDCC/SVM_Calc/MDSA/SVPWM1/vIntp_PWMFOC_CalSec/CalVaVbVc/CalVb ==
  In1 : Inport
  1/2 : Constant  Value=0.5
  Add : Sum  Inputs=+-
  Bus Selector : BusSelector  OutputSignals=Ualpha,Ubeta
  Data Type Conversion : DataTypeConversion  SaturateOnIntegerOverflow=off  RndMeth=Floor
  Data Type Conversion1 : DataTypeConversion  SaturateOnIntegerOverflow=off  RndMeth=Floor
  Data Type Conversion2 : DataTypeConversion  SaturateOnIntegerOverflow=off  RndMeth=Floor
  Product1 : Product
  Product2 : Product
  Sqrt(3)/2 : Constant  Value=0.866025
  Vb : Outport
  wires:
  In1/1 -> Bus Selector/1
  Bus Selector/2 -> Product1/1  "<Ubeta>"
  Add/1 -> Data Type Conversion2/1
  Sqrt(3)/2/1 -> Data Type Conversion/1
  Data Type Conversion/1 -> Product2/2
  1/2/1 -> Data Type Conversion1/1
  Bus Selector/1 -> Product2/1  "<Ualpha>"
  Data Type Conversion1/1 -> Product1/2
  Product2/1 -> Add/1
  Product1/1 -> Add/2
  Data Type Conversion2/1 -> Vb/1

== system MDCC_DeadComp/DoCurCtr_sys/MDCC/SVM_Calc/MDSA/SVPWM1/vIntp_PWMFOC_CalSec/CalVaVbVc/CalVc ==
  In1 : Inport
  -1/2 : Constant  Value=-0.5
  -Sqrt(3)/2 : Constant  Value=-0.866025
  Add : Sum
  Bus Selector : BusSelector  OutputSignals=Ualpha,Ubeta
  Data Type Conversion : DataTypeConversion  SaturateOnIntegerOverflow=off  RndMeth=Floor
  Data Type Conversion1 : DataTypeConversion  SaturateOnIntegerOverflow=off  RndMeth=Floor
  Data Type Conversion2 : DataTypeConversion  SaturateOnIntegerOverflow=off  RndMeth=Floor
  Product1 : Product
  Product2 : Product
  Vc : Outport
  wires:
  In1/1 -> Bus Selector/1
  Bus Selector/2 -> Product1/1  "<Ubeta>"
  Add/1 -> Data Type Conversion2/1
  -Sqrt(3)/2/1 -> Data Type Conversion/1
  Data Type Conversion/1 -> Product2/2
  -1/2/1 -> Data Type Conversion1/1
  Bus Selector/1 -> Product2/1  "<Ualpha>"
  Data Type Conversion1/1 -> Product1/2
  Product2/1 -> Add/1
  Product1/1 -> Add/2
  Data Type Conversion2/1 -> Vc/1

== system MDCC_DeadComp/DoCurCtr_sys/MDCC/SVM_Calc/MDSA/SVPWM1/vIntp_PWMFOC_CalTriCompValue/CalCMPValue/Sec1 ==
  Bus_Tabc_IN : Inport
  Action Port : ActionPort
  Bus Creator1 : BusCreator  Inputs=3
  Bus Selector : BusSelector  OutputSignals=signal2,signal1,signal3
  Signal Conversion : SignalConversion  OverrideOpt=off
  Signal Conversion1 : SignalConversion  OverrideOpt=off
  Signal Conversion2 : SignalConversion  OverrideOpt=off
  Bus_CMP : Outport
  wires:
  Bus_Tabc_IN/1 -> Bus Selector/1
  Bus Creator1/1 -> Bus_CMP/1
  Bus Selector/1 -> Signal Conversion/1  "<signal2>"
  Bus Selector/2 -> Signal Conversion1/1  "<signal1>"
  Bus Selector/3 -> Signal Conversion2/1  "<signal3>"
  Signal Conversion/1 -> Bus Creator1/1
  Signal Conversion1/1 -> Bus Creator1/2
  Signal Conversion2/1 -> Bus Creator1/3

== system MDCC_DeadComp/DoCurCtr_sys/MDCC/SVM_Calc/MDSA/SVPWM1/vIntp_PWMFOC_CalTriCompValue/CalCMPValue/Sec2 ==
  Bus_Tabc_IN : Inport
  Action Port : ActionPort
  Bus Creator : BusCreator  Inputs=3
  Bus Selector : BusSelector  OutputSignals=signal1,signal3,signal2
  Signal Conversion : SignalConversion  OverrideOpt=off
  Signal Conversion1 : SignalConversion  OverrideOpt=off
  Signal Conversion2 : SignalConversion  OverrideOpt=off
  Bus_CMP : Outport
  wires:
  Bus Creator/1 -> Bus_CMP/1
  Bus Selector/1 -> Signal Conversion/1  "<signal1>"
  Bus Selector/2 -> Signal Conversion1/1  "<signal3>"
  Bus Selector/3 -> Signal Conversion2/1  "<signal2>"
  Bus_Tabc_IN/1 -> Bus Selector/1
  Signal Conversion/1 -> Bus Creator/1
  Signal Conversion1/1 -> Bus Creator/2
  Signal Conversion2/1 -> Bus Creator/3

== system MDCC_DeadComp/DoCurCtr_sys/MDCC/SVM_Calc/MDSA/SVPWM1/vIntp_PWMFOC_CalTriCompValue/CalCMPValue/Sec3 ==
  Bus_Tabc_IN : Inport
  Action Port : ActionPort
  Bus Creator : BusCreator  Inputs=3
  Bus Selector : BusSelector  OutputSignals=signal1,signal2,signal3
  Signal Conversion : SignalConversion  OverrideOpt=off
  Signal Conversion1 : SignalConversion  OverrideOpt=off
  Signal Conversion2 : SignalConversion  OverrideOpt=off
  Bus_CMP : Outport
  wires:
  Bus Creator/1 -> Bus_CMP/1
  Bus_Tabc_IN/1 -> Bus Selector/1
  Bus Selector/1 -> Signal Conversion/1  "<signal1>"
  Bus Selector/2 -> Signal Conversion1/1  "<signal2>"
  Bus Selector/3 -> Signal Conversion2/1  "<signal3>"
  Signal Conversion/1 -> Bus Creator/1
  Signal Conversion1/1 -> Bus Creator/2
  Signal Conversion2/1 -> Bus Creator/3

== system MDCC_DeadComp/DoCurCtr_sys/MDCC/SVM_Calc/MDSA/SVPWM1/vIntp_PWMFOC_CalTriCompValue/CalCMPValue/Sec4 ==
  Bus_Tabc_IN : Inport
  Action Port : ActionPort
  Bus Creator : BusCreator  Inputs=3
  Bus Selector : BusSelector  OutputSignals=signal3,signal2,signal1
  Signal Conversion : SignalConversion  OverrideOpt=off
  Signal Conversion1 : SignalConversion  OverrideOpt=off
  Signal Conversion2 : SignalConversion  OverrideOpt=off
  Bus_CMP : Outport
  wires:
  Bus Creator/1 -> Bus_CMP/1
  Bus Selector/1 -> Signal Conversion/1  "<signal3>"
  Bus Selector/2 -> Signal Conversion1/1  "<signal2>"
  Bus Selector/3 -> Signal Conversion2/1  "<signal1>"
  Bus_Tabc_IN/1 -> Bus Selector/1
  Signal Conversion/1 -> Bus Creator/1
  Signal Conversion1/1 -> Bus Creator/2
  Signal Conversion2/1 -> Bus Creator/3

== system MDCC_DeadComp/DoCurCtr_sys/MDCC/SVM_Calc/MDSA/SVPWM1/vIntp_PWMFOC_CalTriCompValue/CalCMPValue/Sec5 ==
  Bus_Tabc_IN : Inport
  Action Port : ActionPort
  Bus Creator : BusCreator  Inputs=3
  Bus Selector : BusSelector  OutputSignals=signal3,signal1,signal2
  Signal Conversion : SignalConversion  OverrideOpt=off
  Signal Conversion1 : SignalConversion  OverrideOpt=off
  Signal Conversion2 : SignalConversion  OverrideOpt=off
  Bus_CMP : Outport
  wires:
  Bus Creator/1 -> Bus_CMP/1
  Bus Selector/1 -> Signal Conversion/1  "<signal3>"
  Bus Selector/2 -> Signal Conversion1/1  "<signal1>"
  Bus Selector/3 -> Signal Conversion2/1  "<signal2>"
  Bus_Tabc_IN/1 -> Bus Selector/1
  Signal Conversion/1 -> Bus Creator/1
  Signal Conversion1/1 -> Bus Creator/2
  Signal Conversion2/1 -> Bus Creator/3

== system MDCC_DeadComp/DoCurCtr_sys/MDCC/SVM_Calc/MDSA/SVPWM1/vIntp_PWMFOC_CalTriCompValue/CalCMPValue/Sec6 ==
  Bus_Tabc_IN : Inport
  Action Port : ActionPort
  Bus Creator : BusCreator  Inputs=3
  Bus Selector : BusSelector  OutputSignals=signal2,signal3,signal1
  Signal Conversion : SignalConversion  OverrideOpt=off
  Signal Conversion1 : SignalConversion  OverrideOpt=off
  Signal Conversion2 : SignalConversion  OverrideOpt=off
  Bus_CMP : Outport
  wires:
  Bus Creator/1 -> Bus_CMP/1
  Bus_Tabc_IN/1 -> Bus Selector/1
  Bus Selector/2 -> Signal Conversion1/1  "<signal3>"
  Bus Selector/3 -> Signal Conversion2/1  "<signal1>"
  Bus Selector/1 -> Signal Conversion/1  "<signal2>"
  Signal Conversion/1 -> Bus Creator/1
  Signal Conversion1/1 -> Bus Creator/2
  Signal Conversion2/1 -> Bus Creator/3

== system MDCC_DeadComp/DoCurCtr_sys/MDCC/SVM_Calc/MDSA/SVPWM1/vIntp_PWMFOC_CalTriCompValue/CalTabc/Cal_T1T2 ==
  Bus_XYZ_IN : Inport
  N_VALUE_IN : Inport  Port=2
  Data Type Conversion : DataTypeConversion  SaturateOnIntegerOverflow=off  RndMeth=Floor
  Merge : Merge  Inputs=6
  Sec1 : Subsystem
  Sec2 : Subsystem
  Sec3 : Subsystem
  Sec4 : Subsystem
  Sec5 : Subsystem
  Sec6 : Subsystem
  Switch Case : SwitchCase  CaseConditions={1,2,3,4,5,6}  ShowDefaultCase=off
  Bus_T1T2_OUT : Outport
  wires:
  Merge/1 -> Bus_T1T2_OUT/1
  N_VALUE_IN/1 -> Data Type Conversion/1
  Bus_XYZ_IN/1 -> Sec5/1(Bus_XYZ_IN), Sec6/1(Bus_XYZ_IN), Sec4/1(Bus_XYZ_IN), Sec3/1(Bus_XYZ_IN), Sec2/1(Bus_XYZ_IN), Sec1/1(Bus_XYZ_IN)
  Data Type Conversion/1 -> Switch Case/1
  Switch Case/1 -> [Cal_T1T2_Sec1]
  Switch Case/2 -> [Cal_T1T2_Sec2]
  Switch Case/3 -> [Cal_T1T2_Sec3]
  Switch Case/4 -> [Cal_T1T2_Sec4]
  Switch Case/5 -> [Cal_T1T2_Sec5]
  Switch Case/6 -> [Cal_T1T2_Sec6]
  [Cal_T1T2_Sec1] -> Sec1/Action
  [Cal_T1T2_Sec3] -> Sec3/Action
  [Cal_T1T2_Sec4] -> Sec4/Action
  [Cal_T1T2_Sec5] -> Sec5/Action
  [Cal_T1T2_Sec6] -> Sec6/Action
  [Cal_T1T2_Sec2] -> Sec2/Action
  Sec4/1(Bus_T1T2) -> Merge/4
  Sec3/1(Bus_T1T2) -> Merge/3
  Sec2/1(Bus_T1T2) -> Merge/2
  Sec5/1(Bus_T1T2) -> Merge/5
  Sec6/1(Bus_T1T2) -> Merge/6
  Sec1/1(Bus_T1T2) -> Merge/1

== system MDCC_DeadComp/DoCurCtr_sys/MDCC/SVM_Calc/MDSA/SVPWM1/vIntp_PWMFOC_CalTriCompValue/CalTabc/Cal_TabcValue ==
  Bus_T1T2_IN : Inport
  Bus_Ts_Vdc : Inport  Port=2
  CalTabcValue : Subsystem
  ManageT1T2 : Subsystem
  Bus_Tabc : Outport
  wires:
  Bus_Ts_Vdc/1 -> CalTabcValue/2(Bus_Ts_Vdc), ManageT1T2/2(Bus_Ts_Vdc)
  Bus_T1T2_IN/1 -> ManageT1T2/1(Bus_T1T2_IN)
  ManageT1T2/1(Bus_T1T2_Adjusted) -> CalTabcValue/1(Bus_T1T2_Adjusted_IN)
  CalTabcValue/1(Bus_Tabc) -> Bus_Tabc/1

== system MDCC_DeadComp/DoCurCtr_sys/MDCC/SVM_Calc/MDSA/SVPWM1/vIntp_PWMFOC_CalTriCompValue/CalXYZ/Cal_X ==
  Bus_UalphaUbeta : Inport
  Bus_Ts_Vdc : Inport  Port=2
  Bus Selector : BusSelector  OutputSignals=Ubeta
  Bus Selector1 : BusSelector  OutputSignals=Ts,Vdc
  Data Type Conversion{,1..4} (5 alike) : DataTypeConversion  SaturateOnIntegerOverflow=off  RndMeth=Floor
  Divide : Product  Inputs=*/
  Product : Product
  Product1 : Product
  Sqrt(3) : Constant  Value=1.7320508
  X_Value : Outport
  wires:
  Bus Selector1/2 -> Data Type Conversion1/1  "<Vdc>"
  Bus Selector1/1 -> Data Type Conversion2/1  "<Ts>"
  Bus_Ts_Vdc/1 -> Bus Selector1/1
  Bus_UalphaUbeta/1 -> Bus Selector/1
  Sqrt(3)/1 -> Data Type Conversion/1
  Divide/1 -> Data Type Conversion3/1
  Product/1 -> Product1/2
  Bus Selector/1 -> Product1/1  "<Ubeta>"
  Product1/1 -> Data Type Conversion4/1
  Data Type Conversion/1 -> Product/2
  Data Type Conversion1/1 -> Divide/2
  Data Type Conversion2/1 -> Divide/1
  Data Type Conversion3/1 -> Product/1
  Data Type Conversion4/1 -> X_Value/1

== system MDCC_DeadComp/DoCurCtr_sys/MDCC/SVM_Calc/MDSA/SVPWM1/vIntp_PWMFOC_CalTriCompValue/CalXYZ/Cal_Y ==
  Bus_UalphaUbeta : Inport
  Bus_Ts_Vdc : Inport  Port=2
  3/2 : Constant  Value=1.5
  Add : Sum
  Bus Selector : BusSelector  OutputSignals=Ualpha,Ubeta
  Bus Selector1 : BusSelector  OutputSignals=Ts,Vdc
  Constant2 : Constant
  Data Type Conversion{,1..6} (7 alike) : DataTypeConversion  SaturateOnIntegerOverflow=off  RndMeth=Floor
  Divide : Product  Inputs=*/
  Divide1 : Product  Inputs=*/  OutDataTypeStr=single
  Product : Product
  Product1 : Product
  Product2 : Product
  Sqrt(3)/2 : Constant  Value=0.866025
  Y_Value : Outport
  wires:
  Bus Selector1/2 -> Data Type Conversion2/1  "<Vdc>"
  Bus Selector1/1 -> Data Type Conversion3/1  "<Ts>"
  Bus_Ts_Vdc/1 -> Bus Selector1/1
  Data Type Conversion6/1 -> Product2/2
  Data Type Conversion5/1 -> Product2/1
  Bus_UalphaUbeta/1 -> Bus Selector/1
  Sqrt(3)/2/1 -> Data Type Conversion/1
  Data Type Conversion/1 -> Product/2
  Bus Selector/2 -> Product/1  "<Ubeta>"
  3/2/1 -> Data Type Conversion1/1
  Data Type Conversion1/1 -> Product1/2
  Bus Selector/1 -> Product1/1  "<Ualpha>"
  Product1/1 -> Add/1
  Product/1 -> Add/2
  Add/1 -> Data Type Conversion5/1
  Data Type Conversion2/1 -> Divide/2
  Data Type Conversion3/1 -> Divide/1
  Divide1/1 -> Data Type Conversion6/1
  Divide/1 -> Divide1/1
  Constant2/1 -> Data Type Conversion4/1
  Product2/1 -> Y_Value/1
  Data Type Conversion4/1 -> Divide1/2

== system MDCC_DeadComp/DoCurCtr_sys/MDCC/SVM_Calc/MDSA/SVPWM1/vIntp_PWMFOC_CalTriCompValue/CalXYZ/Cal_Z ==
  Bus_UalphaUbeta : Inport
  Bus_Ts_Vdc : Inport  Port=2
  3/2 : Constant  Value=1.5
  Add : Sum  Inputs=-+
  Bus Selector : BusSelector  OutputSignals=Ualpha,Ubeta
  Bus Selector1 : BusSelector  OutputSignals=Ts,Vdc
  Constant2 : Constant
  Data Type Conversion{,1..6} (7 alike) : DataTypeConversion  SaturateOnIntegerOverflow=off  RndMeth=Floor
  Divide : Product  Inputs=*/
  Divide1 : Product  Inputs=*/
  Product : Product
  Product1 : Product
  Product2 : Product
  Sqrt(3)/2 : Constant  Value=0.866025
  Z_Value : Outport
  wires:
  Bus Selector1/2 -> Data Type Conversion2/1  "<Vdc>"
  Bus Selector1/1 -> Data Type Conversion3/1  "<Ts>"
  Bus_Ts_Vdc/1 -> Bus Selector1/1
  Data Type Conversion6/1 -> Product2/2
  Data Type Conversion5/1 -> Product2/1
  Data Type Conversion4/1 -> Divide1/2
  Product2/1 -> Z_Value/1
  Constant2/1 -> Data Type Conversion4/1
  Divide/1 -> Divide1/1
  Divide1/1 -> Data Type Conversion6/1
  Data Type Conversion3/1 -> Divide/1
  Data Type Conversion2/1 -> Divide/2
  Add/1 -> Data Type Conversion5/1
  Product/1 -> Add/2
  Product1/1 -> Add/1
  Bus Selector/1 -> Product1/1  "<Ualpha>"
  Data Type Conversion1/1 -> Product1/2
  3/2/1 -> Data Type Conversion1/1
  Bus Selector/2 -> Product/1  "<Ubeta>"
  Data Type Conversion/1 -> Product/2
  Sqrt(3)/2/1 -> Data Type Conversion/1
  Bus_UalphaUbeta/1 -> Bus Selector/1

== system MDCC_DeadComp/DoCurCtr_sys/MDCC/UdUqCalc_Sys/MDCC_MCF_Sys1/Enabled Subsystem/Harmonic_Injection_11/Subsystem/Harm_11Step_KpKi ==
  MCF_Harm_isdDes11 : Inport
  MCF_Harm_isqDes11 : Inport  Port=2
  MCF_Harm_isdAct11 : Inport  Port=3
  MCF_Harm_isqAct11 : Inport  Port=4
  MCF_flgHarm11PIRest : Inport  Port=5
  MCF_Harm11_Kp : Inport  Port=6
  MCF_Harm11_Ki : Inport  Port=7
  Harm_11Step_daxis_PI : Subsystem
  Harm_11Step_qaxis_PI : Subsystem
  MCF_Harm_ud11PI : Outport  VectorParamsAs1DForOutWhenUnconnected=off
  MCF_Harm_uq11PI : Outport  Port=2  VectorParamsAs1DForOutWhenUnconnected=off
  wires:
  MCF_Harm_isqAct11/1 -> Harm_11Step_qaxis_PI/2(MCF_Harm_isqAct11)
  MCF_Harm_isqDes11/1 -> Harm_11Step_qaxis_PI/1(MCF_Harm_isqDes11)
  MCF_Harm_isdAct11/1 -> Harm_11Step_daxis_PI/2(MCF_Harm_isdAct11)
  MCF_Harm11_Ki/1 -> Harm_11Step_qaxis_PI/4(MCF_Harm_Ki), Harm_11Step_daxis_PI/4(MCF_Harm_Ki)
  MCF_Harm11_Kp/1 -> Harm_11Step_qaxis_PI/3(MCF_Harm_Kp), Harm_11Step_daxis_PI/3(MCF_Harm_Kp)
  MCF_Harm_isdDes11/1 -> Harm_11Step_daxis_PI/1(MCF_Harm_isdDes11)
  Harm_11Step_qaxis_PI/1(MCF_Harm_uq11PI) -> MCF_Harm_uq11PI/1  "VfMDCC_MCF_Harm_uq11PI_V"
  Harm_11Step_daxis_PI/1(MCF_Harm_ud11PI) -> MCF_Harm_ud11PI/1  "VfMDCC_MCF_Harm_ud11PI_V"
  MCF_flgHarm11PIRest/1 -> Harm_11Step_daxis_PI/5(MCF_flgHarm11PIRest), Harm_11Step_qaxis_PI/5(MCF_flgHarm11PIRest)

== system MDCC_DeadComp/DoCurCtr_sys/MDCC/UdUqCalc_Sys/MDCC_MCF_Sys1/Enabled Subsystem/Harmonic_Injection_11/Subsystem/RevPark ==
  MCF_Harm_ud11PI : Inport
  MCF_Harm_uq11PI : Inport  Port=2
  MCF_Sin11Ag : Inport  Port=3
  MCF_Cos11Ag : Inport  Port=4
  Add : Sum  Inputs=+-
  Add1 : Sum
  Product{,1..3} (4 alike) : Product
  MCF_uAlpha_Harm11 : Outport  VectorParamsAs1DForOutWhenUnconnected=off
  MCF_uBeta_Harm11 : Outport  Port=2  VectorParamsAs1DForOutWhenUnconnected=off
  wires:
  Product3/1 -> Add1/2
  MCF_Harm_ud11PI/1 -> Product3/1, Product/1
  MCF_Cos11Ag/1 -> Product2/2, Product/2
  Add/1 -> MCF_uAlpha_Harm11/1
  MCF_Sin11Ag/1 -> Product1/2, Product3/2
  Add1/1 -> MCF_uBeta_Harm11/1
  MCF_Harm_uq11PI/1 -> Product2/1, Product1/1
  Product/1 -> Add/1
  Product2/1 -> Add1/1
  Product1/1 -> Add/2

== system MDCC_DeadComp/DoCurCtr_sys/MDCC/UdUqCalc_Sys/MDCC_MCF_Sys1/Enabled Subsystem/Harmonic_Injection_13/Subsystem/Harm_13Step_KpKi ==
  MCF_Harm_isdDes13 : Inport
  MCF_Harm_isqDes13 : Inport  Port=2
  MCF_Harm_isdAct13 : Inport  Port=3
  MCF_Harm_isqAct13 : Inport  Port=4
  MCF_flgHarm13PIRest : Inport  Port=5
  MCF_Harm13_Kp : Inport  Port=6
  MCF_Harm13_Ki : Inport  Port=7
  Harm_13Step_daxis_PI : Subsystem
  Harm_13Step_qaxis_PI : Subsystem
  MCF_Harm_ud13PI : Outport  VectorParamsAs1DForOutWhenUnconnected=off
  MCF_Harm_uq13PI : Outport  Port=2  VectorParamsAs1DForOutWhenUnconnected=off
  wires:
  MCF_Harm_isqAct13/1 -> Harm_13Step_qaxis_PI/2(MCF_Harm_isqAct13)
  MCF_Harm_isqDes13/1 -> Harm_13Step_qaxis_PI/1(MCF_Harm_isqDes13)
  MCF_Harm_isdAct13/1 -> Harm_13Step_daxis_PI/2(MCF_Harm_isdAct13)
  MCF_Harm13_Ki/1 -> Harm_13Step_qaxis_PI/4(MCF_Harm_Ki), Harm_13Step_daxis_PI/4(MCF_Harm_Ki)
  MCF_Harm13_Kp/1 -> Harm_13Step_qaxis_PI/3(MCF_Harm_Kp), Harm_13Step_daxis_PI/3(MCF_Harm_Kp)
  MCF_Harm_isdDes13/1 -> Harm_13Step_daxis_PI/1(MCF_Harm_isdDes13)
  Harm_13Step_qaxis_PI/1(MCF_Harm_uq13PI) -> MCF_Harm_uq13PI/1  "VfMDCC_MCF_Harm_uq13PI_V"
  Harm_13Step_daxis_PI/1(MCF_Harm_ud13PI) -> MCF_Harm_ud13PI/1  "VfMDCC_MCF_Harm_ud13PI_V"
  MCF_flgHarm13PIRest/1 -> Harm_13Step_daxis_PI/5(MCF_flgHarm13PIRest), Harm_13Step_qaxis_PI/5(MCF_flgHarm13PIRest)

== system MDCC_DeadComp/DoCurCtr_sys/MDCC/UdUqCalc_Sys/MDCC_MCF_Sys1/Enabled Subsystem/Harmonic_Injection_13/Subsystem/RevPark ==
  MCF_Harm_ud13PI : Inport
  MCF_Harm_uq13PI : Inport  Port=2
  MCF_Sin13Ag : Inport  Port=3
  MCF_Cos13Ag : Inport  Port=4
  Add : Sum  Inputs=+-
  Add1 : Sum
  Product{,1..3} (4 alike) : Product
  MCF_uAlpha_Harm13 : Outport  VectorParamsAs1DForOutWhenUnconnected=off
  MCF_uBeta_Harm13 : Outport  Port=2  VectorParamsAs1DForOutWhenUnconnected=off
  wires:
  Product3/1 -> Add1/2
  MCF_Harm_ud13PI/1 -> Product3/1, Product/1
  MCF_Cos13Ag/1 -> Product2/2, Product/2
  Add/1 -> MCF_uAlpha_Harm13/1
  MCF_Sin13Ag/1 -> Product1/2, Product3/2
  Add1/1 -> MCF_uBeta_Harm13/1
  MCF_Harm_uq13PI/1 -> Product2/1, Product1/1
  Product/1 -> Add/1
  Product2/1 -> Add1/1
  Product1/1 -> Add/2

== system MDCC_DeadComp/DoCurCtr_sys/MDCC/UdUqCalc_Sys/MDCC_MCF_Sys1/Enabled Subsystem/Harmonic_Injection_5/Subsystem/Harm_5Step_KpKi ==
  MCF_Harm_isdDes5 : Inport
  MCF_Harm_isqDes5 : Inport  Port=2
  MCF_Harm_isdAct5 : Inport  Port=3
  MCF_Harm_isqAct5 : Inport  Port=4
  MCF_flgHarm5PIRest : Inport  Port=5
  MCF_Harm5_Kp : Inport  Port=6
  MCF_Harm5_Ki : Inport  Port=7
  Harm_5Step_daxis_PI : Subsystem
  Harm_5Step_qaxis_PI : Subsystem
  MCF_Harm_ud5PI : Outport  VectorParamsAs1DForOutWhenUnconnected=off
  MCF_Harm_uq5PI : Outport  Port=2  VectorParamsAs1DForOutWhenUnconnected=off
  wires:
  MCF_Harm_isqAct5/1 -> Harm_5Step_qaxis_PI/2(MCF_Harm_isqAct5)
  MCF_Harm_isqDes5/1 -> Harm_5Step_qaxis_PI/1(MCF_Harm_isqDes5)
  MCF_Harm_isdAct5/1 -> Harm_5Step_daxis_PI/2(MCF_Harm_isdAct5)
  MCF_Harm5_Ki/1 -> Harm_5Step_qaxis_PI/4(MCF_Harm_Ki), Harm_5Step_daxis_PI/4(MCF_Harm_Ki)
  MCF_Harm5_Kp/1 -> Harm_5Step_qaxis_PI/3(MCF_Harm_Kp), Harm_5Step_daxis_PI/3(MCF_Harm_Kp)
  MCF_Harm_isdDes5/1 -> Harm_5Step_daxis_PI/1(MCF_Harm_isdDes5)
  Harm_5Step_qaxis_PI/1(MCF_Harm_uq5PI) -> MCF_Harm_uq5PI/1  "VfMDCC_MCF_Harm_uq5PI_V"
  Harm_5Step_daxis_PI/1(MCF_Harm_ud5PI) -> MCF_Harm_ud5PI/1  "VfMDCC_MCF_Harm_ud5PI_V"
  MCF_flgHarm5PIRest/1 -> Harm_5Step_daxis_PI/5(MCF_flgHarm5PIRest), Harm_5Step_qaxis_PI/5(MCF_flgHarm5PIRest)

== system MDCC_DeadComp/DoCurCtr_sys/MDCC/UdUqCalc_Sys/MDCC_MCF_Sys1/Enabled Subsystem/Harmonic_Injection_5/Subsystem/RevPark ==
  MCF_Harm_ud5PI : Inport
  MCF_Harm_uq5PI : Inport  Port=2
  MCF_Sin5Ag : Inport  Port=3
  MCF_Cos5Ag : Inport  Port=4
  Add : Sum  Inputs=+-
  Add1 : Sum
  Product{,1..3} (4 alike) : Product
  MCF_uAlpha_Harm5 : Outport  VectorParamsAs1DForOutWhenUnconnected=off
  MCF_uBeta_Harm5 : Outport  Port=2  VectorParamsAs1DForOutWhenUnconnected=off
  wires:
  Product3/1 -> Add1/2
  MCF_Harm_ud5PI/1 -> Product3/1, Product/1
  MCF_Cos5Ag/1 -> Product2/2, Product/2
  Add/1 -> MCF_uAlpha_Harm5/1
  MCF_Sin5Ag/1 -> Product1/2, Product3/2
  Add1/1 -> MCF_uBeta_Harm5/1
  MCF_Harm_uq5PI/1 -> Product2/1, Product1/1
  Product/1 -> Add/1
  Product2/1 -> Add1/1
  Product1/1 -> Add/2

== system MDCC_DeadComp/DoCurCtr_sys/MDCC/UdUqCalc_Sys/MDCC_MCF_Sys1/Enabled Subsystem/Harmonic_Injection_7/Subsystem/Harm_7Step_KpKi ==
  MCF_Harm_isdDes7 : Inport
  MCF_Harm_isqDes7 : Inport  Port=2
  MCF_Harm_isdAct7 : Inport  Port=3
  MCF_Harm_isqAct7 : Inport  Port=4
  MCF_flgHarm7PIRest : Inport  Port=5
  MCF_Harm7_Kp : Inport  Port=6
  MCF_Harm7_Ki : Inport  Port=7
  Harm_7Step_daxis_PI : Subsystem
  Harm_7Step_qaxis_PI : Subsystem
  MCF_Harm_ud7PI : Outport  VectorParamsAs1DForOutWhenUnconnected=off
  MCF_Harm_uq7PI : Outport  Port=2  VectorParamsAs1DForOutWhenUnconnected=off
  wires:
  MCF_Harm_isqAct7/1 -> Harm_7Step_qaxis_PI/2(MCF_Harm_isqAct7)
  MCF_Harm_isqDes7/1 -> Harm_7Step_qaxis_PI/1(MCF_Harm_isqDes7)
  MCF_Harm_isdAct7/1 -> Harm_7Step_daxis_PI/2(MCF_Harm_isdAct7)
  MCF_Harm7_Ki/1 -> Harm_7Step_qaxis_PI/4(MCF_Harm_Ki), Harm_7Step_daxis_PI/4(MCF_Harm_Ki)
  MCF_Harm7_Kp/1 -> Harm_7Step_qaxis_PI/3(MCF_Harm_Kp), Harm_7Step_daxis_PI/3(MCF_Harm_Kp)
  MCF_Harm_isdDes7/1 -> Harm_7Step_daxis_PI/1(MCF_Harm_isdDes7)
  Harm_7Step_qaxis_PI/1(MCF_Harm_uq7PI) -> MCF_Harm_uq7PI/1  "VfMDCC_MCF_Harm_uq7PI_V"
  Harm_7Step_daxis_PI/1(MCF_Harm_ud7PI) -> MCF_Harm_ud7PI/1  "VfMDCC_MCF_Harm_ud7PI_V"
  MCF_flgHarm7PIRest/1 -> Harm_7Step_daxis_PI/5(MCF_flgHarm7PIRest), Harm_7Step_qaxis_PI/5(MCF_flgHarm7PIRest)

== system MDCC_DeadComp/DoCurCtr_sys/MDCC/UdUqCalc_Sys/MDCC_MCF_Sys1/Enabled Subsystem/Harmonic_Injection_7/Subsystem/RevPark ==
  MCF_Harm_ud7PI : Inport
  MCF_Harm_uq7PI : Inport  Port=2
  MCF_Sin7Ag : Inport  Port=3
  MCF_Cos7Ag : Inport  Port=4
  Add : Sum  Inputs=+-
  Add1 : Sum
  Product{,1..3} (4 alike) : Product
  MCF_uAlpha_Harm7 : Outport  VectorParamsAs1DForOutWhenUnconnected=off
  MCF_uBeta_Harm7 : Outport  Port=2  VectorParamsAs1DForOutWhenUnconnected=off
  wires:
  Product3/1 -> Add1/2
  MCF_Harm_ud7PI/1 -> Product3/1, Product/1
  MCF_Cos7Ag/1 -> Product2/2, Product/2
  Add/1 -> MCF_uAlpha_Harm7/1
  MCF_Sin7Ag/1 -> Product1/2, Product3/2
  Add1/1 -> MCF_uBeta_Harm7/1
  MCF_Harm_uq7PI/1 -> Product2/1, Product1/1
  Product/1 -> Add/1
  Product2/1 -> Add1/1
  Product1/1 -> Add/2

== system MDCC_DeadComp/DoCurCtr_sys/MDCC/UdUqCalc_Sys/MDCC_MCF_Sys1/Enabled Subsystem/Subsystem1/Park11/Subsystem ==
  In1 : Inport
  MCF_dtPWM : Inport  Port=2
  dB_Harm : Inport  Port=3
  Add : Sum
  Add1 : Sum  Inputs=-+
  Add2 : Sum
  Constant1 : Constant  OutDataTypeStr=single
  Constant2 : Constant  Value=2*pi  OutDataTypeStr=single
  Constant4 : Constant  OutDataTypeStr=single
  Divide{,1..3} (4 alike) : Product  Inputs=**
  Divide4 : Product  Inputs=*/
  Unit Delay : UnitDelay  SampleTime=-1  HasFrameUpgradeWarning=on
  Out1 : Outport
  wires:
  Add/1 -> Out1/1, Unit Delay/1
  Divide/1 -> Add/1
  Constant1/1 -> Add1/2
  Add1/1 -> Divide1/1
  Constant2/1 -> Divide2/1
  MCF_dtPWM/1 -> Divide2/2
  dB_Harm/1 -> Divide3/1
  Divide2/1 -> Divide3/2
  Divide3/1 -> Add2/2
  Constant4/1 -> Add2/1, Divide4/1
  Add2/1 -> Divide4/2
  Divide4/1 -> Divide/2, Add1/1
  In1/1 -> Divide1/2
  Divide1/1 -> Add/2
  Unit Delay/1 -> Divide/1
